simulink model "lw2"  (R2022b)
settings: Solver=VariableStepAuto  StartTime=0.0  StopTime=10.0  RelTol=1e-3
settings Model: Creator=Lenovo  LastModifiedBy=Wasif
settings SolverCC: AlgebraicLoopSolver=TrustRegion
settings DataIOCC: ReturnWorkspaceOutputs=off
settings DebuggingCC: UnconnectedInputMsg=warning  UnconnectedOutputMsg=warning  UnconnectedLineMsg=warning  SFMachineParentedDataDiag=warning  ArithmeticOperatorsInVariantConditions=warning
settings ModelReferenceCC: EnableRefExpFcnMdlSchedulingChecks=on
settings SFSimCC: SimUseLocalCustomCode=off  CustomCodeUndefinedFunction=UseInterfaceOnly
settings RTWCC: RTWUseLocalCustomCode=off  DLArmComputeVersion=19.05

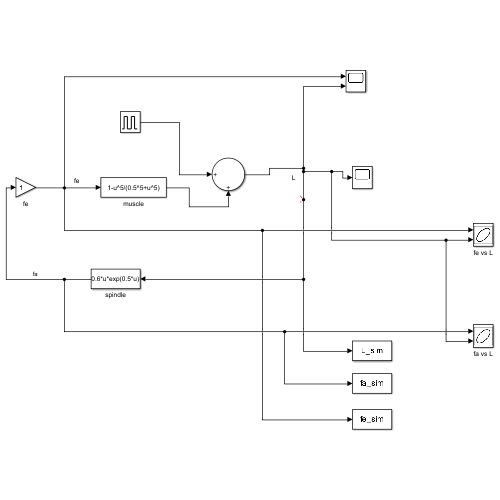
[thumbnail: Simulink's stored preview of the top-level diagram]
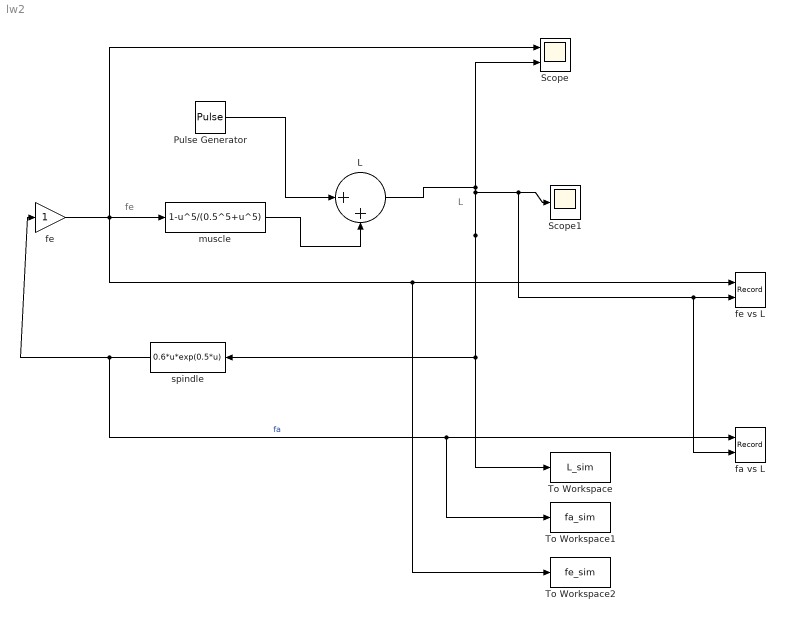
== system lw2 ==
  note: L
  note: fe
  L : Sum  Inputs=|++
  Pulse Generator : DiscretePulseGenerator  PulseType=Time based  Period=15  PulseWidth=0.75
  Scope : Scope  NumInputPorts=2
  Scope1 : Scope
  To Workspace : ToWorkspace  VariableName=L_sim  SampleTime=-1
  To Workspace1 : ToWorkspace  VariableName=fa_sim  SampleTime=-1
  To Workspace2 : ToWorkspace  VariableName=fe_sim  SampleTime=-1
  fa vs L : Record  FileSettingsInternal="{\"entries\":[{\"content\":{\"excelSettings\":{\"content\":{},\"type\":\"Streamout.ExcelSettings\"}},\"type\":\"Streamout.FileSettingStorage\",\"uuid\":\"a1115625-3bc2-4c68-8542-c26aac2bfa5b\"}],\"packageUris\":[\"http://schema.mathworks.com/mf0/streamout_blocks/R2020a\"],\"version\":\"1.0\"}"  Layout=[1 1]  SignalsInternal="{\"entries\":[{\"content\":{\"signals\":[{\"content\":{\"blockPath\":[\"lw2/fa vs L\"],\"channel\":[],\"dimensions\":[1],\"domain\":\"lw2/fa vs L\",\"lineColor\":\"#a2142f\",\"plots\":[1],\"port\":1,\"sid\":[\"\"],\"signalID\":203,\"signalName\":\"fa\"},\"type\":\"RecordBlkView.Signal\",\"uuid\":\"94a7908a-c2ef-42b3-af87-52f9a8039c43\"},{\"content\":{\"blockPath\":[\"lw2/fa vs L\"],\"channel\":[],\"dimensions\":[1],\"domain\":\"lw2/fa vs L\",\"lineColor\":\"#139fff\",\"plots\":[1],\"port\":2,\"sid\":[\"\"],\"signalID\":207,\"signalName\":\"L\"},\"type\":\"RecordBlkView.Signal\",\"uuid\":\"485c7956-47ca-48ea-8bda-e0a2be9f82bf\"}]},\"type\":\"RecordBlkView.InputSignals\",\"uuid\":\"16fbf0eb-4724-4e5f-93c0-23f4bc64947c\"}],\"packageUris\":[\"http://schema.mathworks.com/mf0/streamout_blocks/R2020a\"],\"version\":\"1.0\"}"  VisualizationBindings="{\"xyplotplugin\":{\"info\":[{\"series\":[{\"bindingParametersList\":[{\"parameter\":\"X-Axis\",\"signalID\":203,\"signalName\":\"fa\"},{\"parameter\":\"Y-Axis\",\"signalID\":207,\"signalName\":\"L\"}],\"seriesID\":14368}],\"subplotID\":1}]}}"  CompatibilityTag=XY  st=-1
  fe : Gain
  fe vs L : Record  FileSettingsInternal="{\"entries\":[{\"content\":{\"excelSettings\":{\"content\":{},\"type\":\"Streamout.ExcelSettings\"}},\"type\":\"Streamout.FileSettingStorage\",\"uuid\":\"3712ca67-bfd8-4402-b89c-9305a77dce48\"}],\"packageUris\":[\"http://schema.mathworks.com/mf0/streamout_blocks/R2020a\"],\"version\":\"1.0\"}"  Layout=[1 1]  SignalsInternal="{\"entries\":[{\"content\":{\"signals\":[{\"content\":{\"blockPath\":[\"lw2/fe vs L\"],\"channel\":[],\"dimensions\":[1],\"domain\":\"lw2/fe vs L\",\"lineColor\":\"#a2142f\",\"plots\":[1],\"port\":1,\"sid\":[\"\"],\"signalID\":211,\"signalName\":\"fe\"},\"type\":\"RecordBlkView.Signal\",\"uuid\":\"5ae33130-79f5-4f63-a7d4-21f00fce9ae2\"},{\"content\":{\"blockPath\":[\"lw2/fe vs L\"],\"channel\":[],\"dimensions\":[1],\"domain\":\"lw2/fe vs L\",\"lineColor\":\"#139fff\",\"plots\":[1],\"port\":2,\"sid\":[\"\"],\"signalID\":215,\"signalName\":\"L\"},\"type\":\"RecordBlkView.Signal\",\"uuid\":\"2106560e-d484-45ef-b33e-f48a0ffff06e\"}]},\"type\":\"RecordBlkView.InputSignals\",\"uuid\":\"ce420c11-980e-41f6-8b60-b2e502b83de7\"}],\"packageUris\":[\"http://schema.mathworks.com/mf0/streamout_blocks/R2020a\"],\"version\":\"1.0\"}"  VisualizationBindings="{\"xyplotplugin\":{\"info\":[{\"series\":[{\"bindingParametersList\":[{\"parameter\":\"X-Axis\",\"signalID\":211,\"signalName\":\"fe\"},{\"parameter\":\"Y-Axis\",\"signalID\":215,\"signalName\":\"L\"}],\"seriesID\":4831}],\"subplotID\":1}]}}"  CompatibilityTag=XY  st=-1
  muscle : Fcn  Expr=1-u^5/(0.5^5+u^5)
  spindle : Fcn  Expr=0.6*u*exp(0.5*u)
  wires:
  muscle/1 -> L/2
  Pulse Generator/1 -> L/1
  fe/1 -> Scope/1, To Workspace2/1, fe vs L/1, muscle/1
  L/1 -> To Workspace/1, spindle/1, fa vs L/2, fe vs L/2, Scope1/1, Scope/2
  spindle/1 -> To Workspace1/1, fa vs L/1, fe/1  "fa"
